simulink model "FOC_simulation"  (R2021a)
settings: Solver=ode8  StartTime=0.0  StopTime=6  FixedStep=.001  RelTol=1e-3
InitFcn:
  | params
values from neighbouring files (symbols this model uses):
  A = diag([7 7 7])    [params.m]
  g = 9.81    [params.m]
  J = diag([1 1 1])    [params.m]
  K1 = diag([50 50 50])    [params.m]
  K1_pid = diag([70 70 70])    [params.m]
  K2 = diag([10 10 10])    [params.m]
  K2_pid = diag([20 20 20])    [params.m]
  k3 = diag([30 30 30])    [params.m]
  K3_pid = diag([1 1 1])    [params.m]
  k4 = diag([10 10 10])    [params.m]
  komega = diag([10 10 10])    [params.m]
  kR = diag([50 50 50])    [params.m]
  m = 1    [params.m]
libraries: sharedtransform x3, fod x3, aerolibconvert2 x2
settings Model: Creator=Alejandro Fl  LastModifiedBy=Alejandro Fl

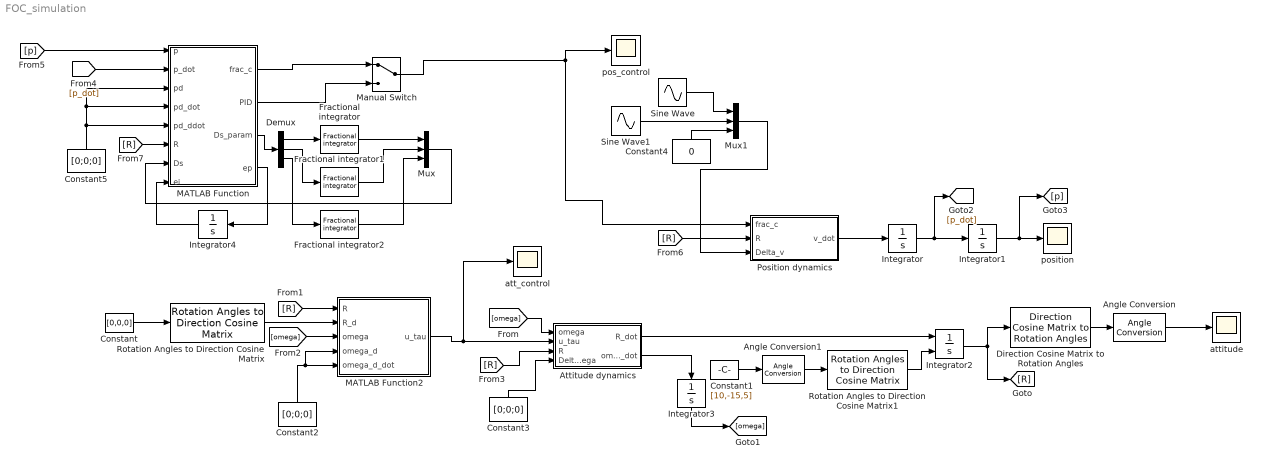
== system FOC_simulation ==
  Angle Conversion : aerolibconvert2/Angle Conversion  IU=rad  OU=deg
  Angle Conversion1 : aerolibconvert2/Angle Conversion  IU=deg  OU=rad
  Attitude dynamics : MATLAB Function  TreatAsAtomicUnit=on
  Constant : Constant  Value=[0,0,0]
  Constant1 : Constant  Value=[10,-15,5]
  Constant2 : Constant  Value=[0;0;0]
  Constant3 : Constant  Value=[0;0;0]
  Constant4 : Constant  Value=0
  Constant5 : Constant  Value=[0;0;0]
  Demux : Demux  Outputs=3
  Direction Cosine Matrix to Rotation Angles : sharedtransform/Direction Cosine Matrix to Rotation Angles  rotationOrder=ZYX  aMode=aMode  action=None  tolerance=eps(2)
      settings: SourceProductBaseCode=AE,PW,DR,MT,UV,VE
  Fractional integrator : fod/Fractional integrator  gam=orden  ww=[0.001; 1000]  n=5  nFod=off
      settings: SourceProductName=FOMCON Toolbox
  Fractional integrator1 : fod/Fractional integrator  gam=orden  ww=[0.001; 1000]  n=5  nFod=off
      settings: SourceProductName=FOMCON Toolbox
  Fractional integrator2 : fod/Fractional integrator  gam=orden  ww=[0.001; 1000]  n=5  nFod=off
      settings: SourceProductName=FOMCON Toolbox
  Integrator : Integrator  InitialCondition=[0;0;0]
  Integrator1 : Integrator  InitialCondition=[2;-1;1.5]
  Integrator2 : Integrator  InitialConditionSource=external
  Integrator3 : Integrator  InitialCondition=[0;0;0]
  Integrator4 : Integrator  InitialCondition=[0;0;0]  LimitOutput=on  UpperSaturationLimit=10  LowerSaturationLimit=-10
  MATLAB Function : MATLAB Function  TreatAsAtomicUnit=on
  MATLAB Function2 : MATLAB Function  TreatAsAtomicUnit=on
  Manual Switch : ManualSwitch
  Mux : Mux  Inputs=3
  Mux1 : Mux  Inputs=3
  Position dynamics : MATLAB Function  TreatAsAtomicUnit=on
  Rotation Angles to Direction Cosine Matrix : sharedtransform/Rotation Angles to Direction Cosine Matrix  rotationOrder=ZYX  aMode=aMode
      settings: SourceProductBaseCode=AE,PW,DR,MT,UV,VE
  Rotation Angles to Direction Cosine Matrix1 : sharedtransform/Rotation Angles to Direction Cosine Matrix  rotationOrder=ZYX  aMode=aMode
      settings: SourceProductBaseCode=AE,PW,DR,MT,UV,VE
  Sine Wave : Sin  Amplitude=20  SampleTime=0
  Sine Wave1 : Sin  Amplitude=30  Frequency=2  SampleTime=0
  att_control : Scope
  attitude : Scope
  pos_control : Scope
  position : Scope
  wires:
  Position dynamics/1(v_dot) -> Integrator/1
  Integrator/1 -> [p_dot], Integrator1/1
  Integrator1/1 -> [p], position/1
  Attitude dynamics/1(R_dot) -> Integrator2/1
  Integrator2/1 -> Direction Cosine Matrix to Rotation Angles/1, [R]
  Attitude dynamics/2(omega_dot) -> Integrator3/1
  Integrator3/1 -> [omega]
  [omega] -> Attitude dynamics/1(omega)
  MATLAB Function2/1(u_tau) -> att_control/1, Attitude dynamics/2(u_tau)
  [R] -> MATLAB Function2/1(R)
  Rotation Angles to Direction Cosine Matrix/1 -> MATLAB Function2/2(R_d)
  Constant/1 -> Rotation Angles to Direction Cosine Matrix/1
  Constant1/1 -> Angle Conversion1/1
  Rotation Angles to Direction Cosine Matrix1/1 -> Integrator2/2
  [omega] -> MATLAB Function2/3(omega)
  Constant2/1 -> MATLAB Function2/5(omega_d_dot), MATLAB Function2/4(omega_d)
  [R] -> Attitude dynamics/3(R)
  Constant3/1 -> Attitude dynamics/4(Delta_omega)
  Direction Cosine Matrix to Rotation Angles/1 -> Angle Conversion/1
  Angle Conversion/1 -> attitude/1
  Angle Conversion1/1 -> Rotation Angles to Direction Cosine Matrix1/1
  Mux1/1 -> Position dynamics/3(Delta_v)
  Manual Switch/1 -> Position dynamics/1(frac_c), pos_control/1
  Constant5/1 -> MATLAB Function/5(pd_ddot), MATLAB Function/4(pd_dot), MATLAB Function/3(pd)
  [p_dot] -> MATLAB Function/2(p_dot)
  [p] -> MATLAB Function/1(p)
  MATLAB Function/3(Ds_param) -> Demux/1
  Demux/1 -> Fractional integrator/1
  Fractional integrator/1 -> Mux/1
  Demux/2 -> Fractional integrator1/1
  Fractional integrator1/1 -> Mux/2
  Demux/3 -> Fractional integrator2/1
  Fractional integrator2/1 -> Mux/3
  Mux/1 -> MATLAB Function/7(Ds)
  [R] -> Position dynamics/2(R)
  [R] -> MATLAB Function/6(R)
  Constant4/1 -> Mux1/3
  MATLAB Function/4(ep) -> Integrator4/1
  Integrator4/1 -> MATLAB Function/8(ei)
  MATLAB Function/1(frac_c) -> Manual Switch/1
  MATLAB Function/2(PID) -> Manual Switch/2
  Sine Wave/1 -> Mux1/1
  Sine Wave1/1 -> Mux1/2

== matlab function FOC_simulation/Attitude dynamics ==
  data: R_dot output; omega_dot output size=[3 1]; omega input size=[3 1]; J parameter size=[3 3]; u_tau input size=[3 1]; R input size=[3 3]; Delta_omega input size=[3 1]
function [R_dot, omega_dot] = fcn(omega,J, u_tau, R, Delta_omega)

omega_hat = [0 -omega(3) omega(2);
             omega(3) 0 -omega(1);
             -omega(2) omega(1) 0];
R_dot = R*omega_hat;
omega_dot = -J\(cross(omega,J*omega)) + J\u_tau + Delta_omega;

== matlab function FOC_simulation/Position dynamics ==
  data: v_dot output size=[3 1]; frac_c input size=[3 1]; R input size=[3 3]; Delta_v input size=[3 1]; g parameter size=1; e3 parameter size=[3 1]; m parameter size=1
function v_dot = fcn(frac_c,R,Delta_v, g, e3, m)

v_dot = -g*e3 + (1/m)*R*frac_c + Delta_v;

== matlab function FOC_simulation/MATLAB Function2 ==
  data: J parameter size=[3 3]; R input size=[3 3]; R_d input size=[3 3]; u_tau output size=[3 1]; omega input size=[3 1]; omega_d input size=[3 1]; omega_d_dot input size=[3 1]; kR parameter size=[3 3]; komega parameter size=[3 3]; k3 parameter size=[3 3]; k4 parameter size=[3 3]
function u_tau = fcn(J, R, R_d, omega, omega_d, omega_d_dot,kR, komega, k3, k4)

omega_hat = [0 -omega(3) omega(2);
             omega(3) 0 -omega(1);
             -omega(2) omega(1) 0];
         
R_er = R_d'*R;
err_R = (R_er - R_er')/2;

e_R = [err_R(3,2); err_R(1,3); err_R(2,1)];
e_omega = omega - R_er'*omega_d;

v_R = [(abs(e_R(1))^(1/2)) * sign(e_R(1));
       (abs(e_R(2))^(1/2)) * sign(e_R(2));
       (abs(e_R(3))^(1/2)) * sign(e_R(3))];

v_omega = [(abs(e_omega(1))^(1/2)) * sign(e_omega(1));
       (abs(e_omega(2))^(1/2)) * sign(e_omega(2));
       (abs(e_omega(3))^(1/2)) * sign(e_omega(3))];


u_tau = -J*(kR*e_R + komega*e_omega + k3*v_R + k4*v_omega) + cross(omega,J*omega) - J*(omega_hat*R_er'*omega_d - R_er'*omega_d_dot);

== matlab function FOC_simulation/MATLAB Function ==
  data: p input size=[3 1]; p_dot input size=[3 1]; pd input size=[3 1]; pd_dot input size=[3 1]; pd_ddot input size=[3 1]; K1 parameter size=[3 3]; K2 parameter size=[3 3]; e3 parameter size=[3 1]; A parameter size=[3 3]; g parameter size=1; R input size=[3 3]; frac_c output size=[3 1]; PID output size=[3 1]; Ds input size=[3 1]; Ds_param output size=[3 1]; m parameter size=1; ei input size=[3 1]; ep output size=[3 1]; K3_pid parameter size=[3 3]; K2_pid parameter size=[3 3]; K1_pid parameter size=[3 3]
function [frac_c,PID,Ds_param,ep] = fcn(p,p_dot,pd,pd_dot,pd_ddot,K1, K2, e3, A, g,R,Ds, m,ei,K3_pid,K2_pid, K1_pid)

ep = p - pd;
ev = p_dot - pd_dot;

s = ev + A*ep;
Ds_param = [abs(s(1))^(1/2) * sign(s(1));
            abs(s(2))^(1/2) * sign(s(2));
            abs(s(3))^(1/2) * sign(s(3))];



frac_c = R \ (m*(-K1*Ds - K2*s + g*e3 + pd_ddot - A*ev));

PID = R \ (m*(-K1_pid*ep - K2_pid*ev -K3_pid*ei + g*e3 + pd_ddot));
